simulink model "linearActuator"  (R2023a)
settings: Solver=FixedStepAuto  StartTime=0.0  StopTime=inf  FixedStep=Ts  RelTol=1e-3
InitFcn:
  | Ts=0.001;
  | set_param('linearActuator/enableDrive','Value','0');
  | load('commandSignals.mat');
libraries: slrealtimeethercatlib x8, simulink x3, dspsigops x1
settings Model: Creator=Wave User  LastModifiedBy=Wave User
settings SolverCC: ConcurrentTasks=on  PositivePriorityOrder=on
settings DataIOCC: ExternalInput=commandSigs.getElement(1),commandSigs.getElement(2),commandSigs.getElement(3)  LoadExternalInput=on
settings OptimizationCC: BlockReduction=off  OptimizeBlockIOStorage=off
settings DebuggingCC: TasksWithSamePriorityMsg=none
settings HardwareCC: ProdBitPerLong=64  ProdLongLongMode=on  ProdHWDeviceType=Intel->x86-64 (Linux 64)
settings RTWCC: Description=Simulink Real-Time  SystemTargetFile=slrealtime.tlc  TemplateMakefile=slrealtime_default_tmf  Toolchain=Simulink Real-Time Toolchain  BuildConfiguration=Faster Runs  CodeExecutionProfiling=on  TargetLang=C++

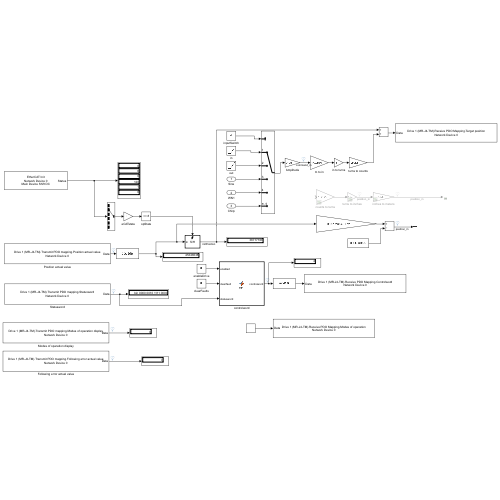
[thumbnail: Simulink's stored preview of the top-level diagram]
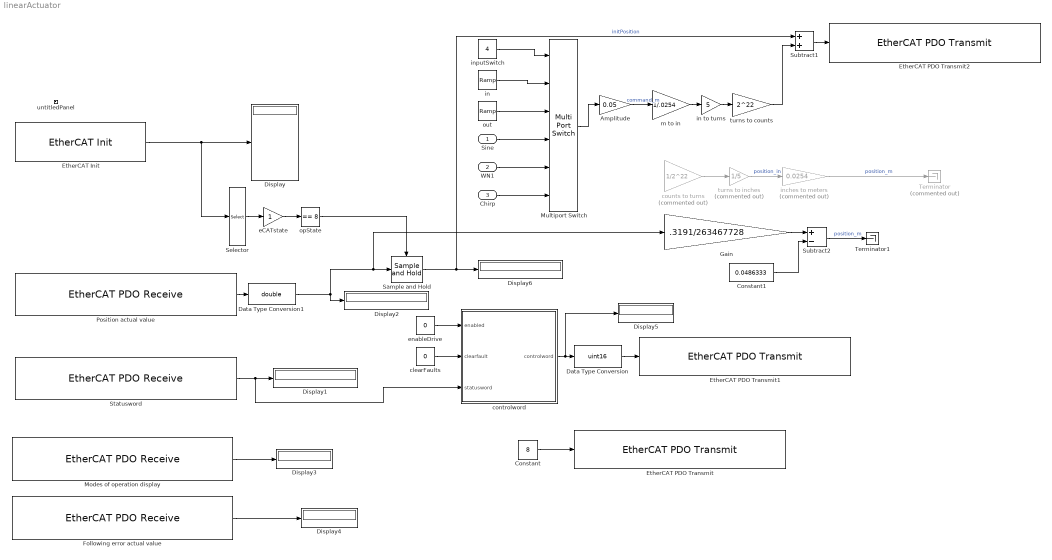
== system linearActuator ==
  Sine : Inport
  WN1 : Inport  Port=2
  Chirp : Inport  Port=3
  Amplitude : Gain  Gain=0.05
  Constant : Constant  Value=8  OutDataTypeStr=int8
  Constant1 : Constant  Value=0.0486333
  Data Type Conversion : DataTypeConversion  OutDataTypeStr=uint16  SaturateOnIntegerOverflow=off  RndMeth=Floor
  Data Type Conversion1 : DataTypeConversion  OutDataTypeStr=double  SaturateOnIntegerOverflow=off  RndMeth=Floor
  Display{,1..6} (7 alike) : Display
      Display1 settings: Format=binary (Stored Integer)
  EtherCAT Init : slrealtimeethercatlib/EtherCAT Init  Priority=0  config_file=C:\Software\linear-actuator\Simulink\linear_actuator.xml  device_id=0  portnum=1  initstate=2  dctuning=0  enaDebug=0  logFile='c:\dbglog.txt'  sample_time=0.001000  DCMode=2
  EtherCAT PDO Transmit : slrealtimeethercatlib/EtherCAT PDO Transmit  Priority=3  sig_name=Drive 1 (MR-J4-TM).Receive PDO Mapping.Modes of operation  sig_offset=568  sig_type=int8  type_size=8  sig_dim=1  device_id=0  sample_time=0.001000
  EtherCAT PDO Transmit1 : slrealtimeethercatlib/EtherCAT PDO Transmit  Priority=3  sig_name=Drive 1 (MR-J4-TM).Receive PDO Mapping.Controlword  sig_offset=576  sig_type=uint16  type_size=16  sig_dim=1  device_id=0  sample_time=0.001000
  EtherCAT PDO Transmit2 : slrealtimeethercatlib/EtherCAT PDO Transmit  Priority=3  sig_name=Drive 1 (MR-J4-TM).Receive PDO Mapping.Target position  sig_offset=640  sig_type=int32  type_size=32  sig_dim=1  device_id=0  sample_time=0.001000
  Following error actual value : slrealtimeethercatlib/EtherCAT PDO Receive  Priority=2  sig_name=Drive 1 (MR-J4-TM).Transmit PDO mapping.Following error actual value  sig_offset=704  sig_type=int32  type_size=32  sig_dim=1  device_id=0  sample_time=0.001000
  Gain : Gain  Gain=.3191/263467728
  Modes of operation display : slrealtimeethercatlib/EtherCAT PDO Receive  Priority=2  sig_name=Drive 1 (MR-J4-TM).Transmit PDO mapping.Modes of operation display  sig_offset=568  sig_type=int8  type_size=8  sig_dim=1  device_id=0  sample_time=0.001000
  Multiport Switch : MultiPortSwitch  Inputs=5  SaturateOnIntegerOverflow=off  InputSameDT=off
  Position actual value : slrealtimeethercatlib/EtherCAT PDO Receive  Priority=2  sig_name=Drive 1 (MR-J4-TM).Transmit PDO mapping.Position actual value  sig_offset=640  sig_type=int32  type_size=32  sig_dim=1  device_id=0  sample_time=0.001000
  Sample and Hold : dspsigops/Sample and Hold  trig=Rising edge  initCond=0  latchinput=off
  Selector : Selector  InputPortWidth=6  IndexOptions=Index vector (dialog)  Indices=[2]  OutputSizes=1
  Statusword : slrealtimeethercatlib/EtherCAT PDO Receive  Priority=2  sig_name=Drive 1 (MR-J4-TM).Transmit PDO mapping.Statusword  sig_offset=576  sig_type=uint16  type_size=16  sig_dim=1  device_id=0  sample_time=0.001000
  Subtract1 : Sum  OutDataTypeStr=int32
  Subtract2 : Sum  Inputs=+-
  Terminator : Terminator  Commented=on
  Terminator1 : Terminator
  clearFaults : Constant  Value=0
  controlword : MATLAB Function  TreatAsAtomicUnit=on
  counts to turns : Gain  Commented=on  Gain=1/2^22
  eCATstate : Gain
  enableDrive : Constant  Value=0
  in : simulink/Sources/Ramp  slope=1/5  start=20  InitialOutput=0
  in to turns : Gain  Gain=5
  inches to meters : Gain  Commented=on  Gain=0.0254
  inputSwitch : Constant  Value=4
  m to in : Gain  Gain=1/.0254
  opState : simulink/Logic and Bit Operations/Compare To Constant  relop===  const=8  OutDataTypeStr=boolean
  out : simulink/Sources/Ramp  slope=-1/5  start=20  InitialOutput=0
  turns to counts : Gain  Gain=2^22
  turns to inches : Gain  Commented=on  Gain=1/5
  untitledPanel : Subsystem  Tag=HiddenForWebPanel  IsWebBlockPanel=on
  wires:
  EtherCAT Init/1 -> Selector/1, Display/1
  Statusword/1 -> controlword/3(statusword), Display1/1
  Modes of operation display/1 -> Display3/1
  Constant/1 -> EtherCAT PDO Transmit/1
  clearFaults/1 -> controlword/2(clearfault)
  enableDrive/1 -> controlword/1(enabled)
  controlword/1(controlword) -> Display5/1, Data Type Conversion/1
  Data Type Conversion/1 -> EtherCAT PDO Transmit1/1
  Following error actual value/1 -> Display4/1
  Selector/1 -> eCATstate/1
  eCATstate/1 -> opState/1
  opState/1 -> Sample and Hold/Trigger
  Sample and Hold/1 -> Display6/1, Subtract1/1  "initPosition"
  Position actual value/1 -> Data Type Conversion1/1
  in/1 -> Multiport Switch/2
  Subtract1/1 -> EtherCAT PDO Transmit2/1
  counts to turns/1 -> turns to inches/1
  turns to inches/1 -> inches to meters/1  "position_in"
  inches to meters/1 -> Terminator/1  "position_m"
  out/1 -> Multiport Switch/3
  inputSwitch/1 -> Multiport Switch/1
  turns to counts/1 -> Subtract1/2
  in to turns/1 -> turns to counts/1
  m to in/1 -> in to turns/1
  Multiport Switch/1 -> Amplitude/1
  Sine/1 -> Multiport Switch/4
  Amplitude/1 -> m to in/1  "command_m"
  WN1/1 -> Multiport Switch/5
  Data Type Conversion1/1 -> Gain/1, Sample and Hold/1, Display2/1
  Chirp/1 -> Multiport Switch/6
  Gain/1 -> Subtract2/1
  Constant1/1 -> Subtract2/2
  Subtract2/1 -> Terminator1/1  "position_m"

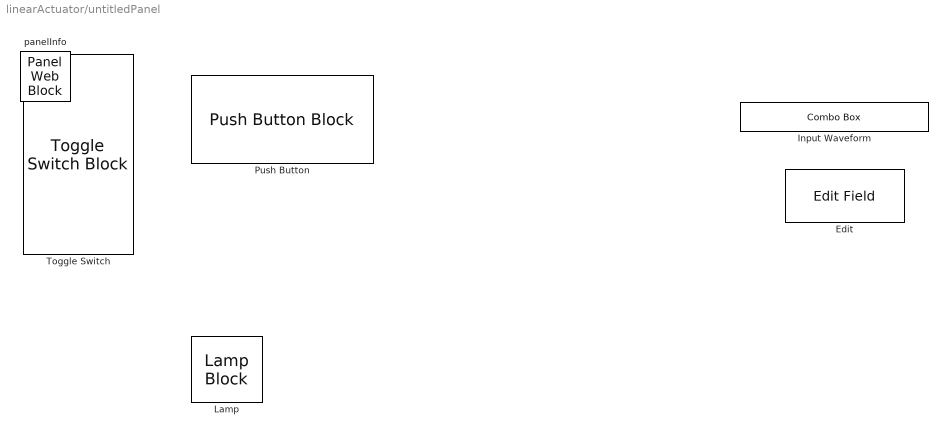
== system linearActuator/untitledPanel ==
  Edit : EditField  Tag=HiddenForWebPanel  PanelInfo="{\"height\":53,\"left\":751,\"panelId\":\"panelId-8f50dd30-35b9-4a99-bcae-21d1638129a7\",\"top\":112,\"type\":\"panelChild\",\"version\":\"2019b\",\"width\":119,\"zIndex\":1500010}"  ShowInitialText=on  Alignment=Center
  Input Waveform : ComboBox  Tag=HiddenForWebPanel  PanelInfo="{\"height\":29,\"left\":735,\"panelId\":\"panelId-8f50dd30-35b9-4a99-bcae-21d1638129a7\",\"top\":66,\"type\":\"panelChild\",\"version\":\"2019b\",\"width\":188,\"zIndex\":1500008}"  LabelPosition=Hide  SelectedLabel=WN1
      settings: Values={{'in', 'out', 'sine', 'WN1', 'Chirp'}, [1 2 3 4 5]}
  Lamp : LampBlock  Tag=HiddenForWebPanel  PanelInfo="{\"height\":66,\"left\":186,\"panelId\":\"panelId-8f50dd30-35b9-4a99-bcae-21d1638129a7\",\"top\":300,\"type\":\"panelChild\",\"version\":\"2019b\",\"width\":71,\"zIndex\":1500006}"  LabelPosition=Hide
  Push Button : PushButtonBlock  Tag=HiddenForWebPanel  PanelInfo="{\"height\":177,\"left\":59,\"panelId\":\"panelId-8f50dd30-35b9-4a99-bcae-21d1638129a7\",\"top\":51,\"type\":\"panelChild\",\"version\":\"2019b\",\"width\":366,\"zIndex\":1500004}"  ButtonText=Clear Faults  OffValue=0.000000
  Toggle Switch : ToggleSwitchBlock  Tag=HiddenForWebPanel  PanelInfo="{\"height\":402,\"left\":469,\"panelId\":\"panelId-8f50dd30-35b9-4a99-bcae-21d1638129a7\",\"top\":65,\"type\":\"panelChild\",\"version\":\"2019b\",\"width\":221,\"zIndex\":1500002}"
      settings: Values={{'Off', 'On'}, [0 1]}
  panelInfo : PanelWebBlock  Tag=HiddenForWebPanel  PanelInfo="{\"compacted\":false,\"height\":649,\"isActiveTab\":true,\"labels\":{},\"left\":726,\"name\":\"Panel\",\"panelId\":\"panelId-8f50dd30-35b9-4a99-bcae-21d1638129a7\",\"tabIndex\":0,\"tabbedSetId\":\"tabbedSet2785537506\",\"top\":272,\"type\":\"panel\",\"version\":\"2019b\",\"visible\":true,\"width\":979,\"zIndex\":1500002}"  PanelSnapshot=<binary blob, 36844 chars, not shown>

== matlab function linearActuator/controlword ==
  data: enabled input; clearfault input; statusword input; controlword output
function controlword = fcn(enabled, clearfault, statusword)

bitstatus = bitget(statusword,1:16);

if ~clearfault
    if enabled
        if bitstatus(1) == 0 % Ready to switch on not ready
            controlword = 6; % command ready switch on
        elseif ~bitstatus(2) % switched not yet on
            controlword = 7; % command switch on
        elseif ~bitstatus(3) % operation not yet enabled
            controlword = 15; % command enable
        else
            controlword = 15; % maintain enabled state
        end
    else
        controlword = 4; % command disabled
    end
else
    controlword = 128; % command clear faults
end
